simulink model "Level4"  (R2012b)
settings: Solver=FixedStepDiscrete  StartTime=0.0  StopTime=50  RelTol=1e-3
InitFcn:
  | N=256;
  | Fs = 1000;
  | bw = 5.6;
undefined symbols (not defined in the file): gcbh, rmidispblock
settings Model: RequirementInfo={'other' '..\..\..\requirements\ebd_srs.doc' '?Simulink_requirement_level4' 'true' 'Simulink_requirement_level4' '' } %GIDa_1821195c_588b_4139_9a4e_c5097c760e25  Creator=aanantha  LastModifiedBy=klindqvi
settings DataIOCC: SaveFormat=Structure  SignalLoggingSaveFormat=ModelDataLogs  SaveOutput=off  SaveTime=off  SignalLoggingName=logsOut
settings OptimizationCC: InlineParams=on  OptimizeModelRefInitCode=on  LifeSpan=1
settings DebuggingCC: ReadBeforeWriteMsg=DisableAll  WriteAfterWriteMsg=DisableAll  WriteAfterReadMsg=DisableAll  SolverPrmCheckMsg=none  InheritedTsInSrcMsg=none  ParameterPrecisionLossMsg=none  FcnCallInpInsideContextMsg=EnableAllAsWarning
settings HardwareCC: ProdLargestAtomicInteger=Long  ProdLargestAtomicFloat=Double  ProdEndianess=LittleEndian  ProdHWDeviceType=ARM Compatible->ARM Cortex
settings RTWCC: SystemTargetFile=ert.tlc  TemplateMakefile=ert_default_tmf  Description=Embedded Coder  GenerateReport=on  RTWVerbose=off  ProcessScript=ert_make_rtw_hook  IncludeHyperlinkInReport=on  LaunchReport=on  PortableWordSizes=on  CodeProfilingSaveOptions=AllData  GenerateTraceInfo=on  GenerateTraceReportSl=on  GenerateTraceReportSf=on  GenerateTraceReportEml=on  GenerateCodeMetricsReport=on
settings CodeAppCC: IgnoreCustomStorageClasses=off
settings ERTTargetCC: CodeReplacementLibrary=GCC ARM Cortex-A8  MultiwordLength=2048  GenerateSampleERTMain=on  ERTCustomFileTemplate=example_file_process.tlc  ConvertIfToSwitch=off  SuppressUnreachableDefaultCases=off

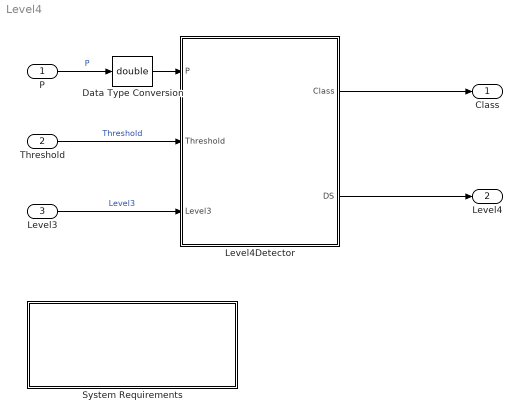
== system Level4 ==
  P : Inport  OutDataTypeStr=single  PortDimensions=1  SampleTime=[0.08900000000000001,0]
  Threshold : Inport  Port=2  OutDataTypeStr=double  PortDimensions=1  SampleTime=[0.08900000000000001,0]
  Level3 : Inport  Port=3  OutDataTypeStr=boolean  PortDimensions=1  SampleTime=[0.08900000000000001,0]
  Data Type Conversion : DataTypeConversion  OutDataTypeStr=double
  Level4Detector : Subsystem
  System Requirements : Subsystem  LoadFcn=rmidispblock('load',gcbh)  mask(System Requirements){id=SystemReq, title=System Requirements}
      mask prompts: title "Block Title"
      mask help: Lists the requirements for the current model.
      mask init:
      | id = 'SystemReq';
      | [w,h] = rmidispblock('display',gcbh);
      settings: CopyFcn=rmidispblock('create',gcbh)  DeleteFcn=rmidispblock('delete',gcbh)  ModelCloseFcn=rmidispblock('close',gcbh)  PreSaveFcn=rmidispblock('close',gcbh)  PostSaveFcn=rmidispblock('open',gcbh)  OpenFcn=rmidispblock('open',gcbh)  MoveFcn=rmidispblock('move',gcbh)
      mask Help: helpview(fullfile(docroot,'toolbox','slvnv','slvnv.map'),'systemrequirements')
      mask Display: text(w/2,h-4,rmidispblock('title',gcbh),'horizontalAlignment','center','verticalAlignment','top')
  Class : Outport  OutDataTypeStr=boolean  PortDimensions=1  SampleTime=[0.08900000000000001,0]
  Level4 : Outport  Port=2  OutDataTypeStr=double  PortDimensions=1  SampleTime=[0.08900000000000001,0]
  wires:
  P/1 -> Data Type Conversion/1  "P"
  Threshold/1 -> Level4Detector/2(Threshold)  "Threshold"
  Level3/1 -> Level4Detector/3(Level3)  "Level3"
  Level4Detector/1(Class) -> Class/1
  Level4Detector/2(DS) -> Level4/1
  Data Type Conversion/1 -> Level4Detector/1(P)

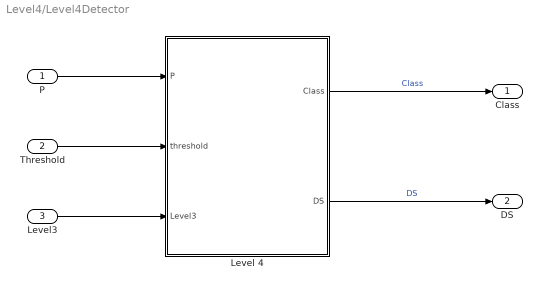
== system Level4/Level4Detector ==
  P : Inport
  Threshold : Inport  Port=2
  Level3 : Inport  Port=3
  Level 4 : MATLAB Function  RequirementInfo={'other' '..\..\requirements\ebd_srs.doc' '@Simulink_requirement_item_8' 'true' 'Simulink_requirement_item_8' 'Requirement' } %GIDa_a0410a00_8e4c_4157_9566_e5717b12b6f9  TreatAsAtomicUnit=on
  Class : Outport
  DS : Outport  Port=2
  wires:
  Level 4/2(DS) -> DS/1  "DS"
  P/1 -> Level 4/1(P)
  Level3/1 -> Level 4/3(Level3)
  Threshold/1 -> Level 4/2(threshold)
  Level 4/1(Class) -> Class/1  "Class"

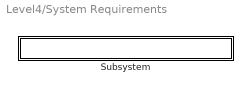
== system Level4/System Requirements ==
  Subsystem : Subsystem  mask{label=0, index=1}
      mask init:
      | label = rmidispblock('label',index);
      settings: OpenFcn=rmidispblock('openReq',gcbh);
      mask Display: text(0,0,label,'horizontalAlignment','left','verticalAlignment','bottom')

== system Level4/System Requirements/Subsystem ==

== matlab function Level4/Level4Detector/Level 4 ==
  data: P input; Class output boolean; DS output; threshold input; Level3 input
function [Class,DS] = Level4Detector(P, threshold, Level3) %#codegen

% Maintain running Noise and Signal History
persistent Noise Signal sCount nCount

% Gains for initializing the Signal/Noise History
initSignalLevelGain = 1;
initNoiseLevelGain = 0.3;


if isempty(Noise)
    % Noise Level
    Noise = P * initNoiseLevelGain;
    nCount = 1;
end

if isempty(Signal)
    % Signal Level
    Signal = P * initSignalLevelGain;
    sCount = 1;
end

DS = (P-Noise)/(Signal-Noise);

% Limit Value of Detection Strength to between 0 and 1
if DS > 1
    DS = 1;
elseif DS <0
    DS = 0;
end

% Update Signal/Noise Histories
if Level3 || (DS>threshold)% if Level 3 detects a-beat; output a-Beat and update signal history
    % Classify as Signal and update Signal History
    Class = true; %boolean(1);  % a-Beat
    Signal = (Signal*sCount + P) / (sCount+1);
    sCount = sCount + 1;
else
    % Classify as Noise and update Noise History
    Class = false; % not-a-Beat
    Noise = (Noise*nCount + P) / (nCount+1);
    nCount = nCount + 1;
end
